simulink model "simulation"  (R2018a)
settings: Solver=VariableStepAuto  StartTime=0.0  StopTime=5  RelTol=1e-3
libraries: simulink x3, vrlib x1
settings Model: Creator=Juan  LastModifiedBy=Juan

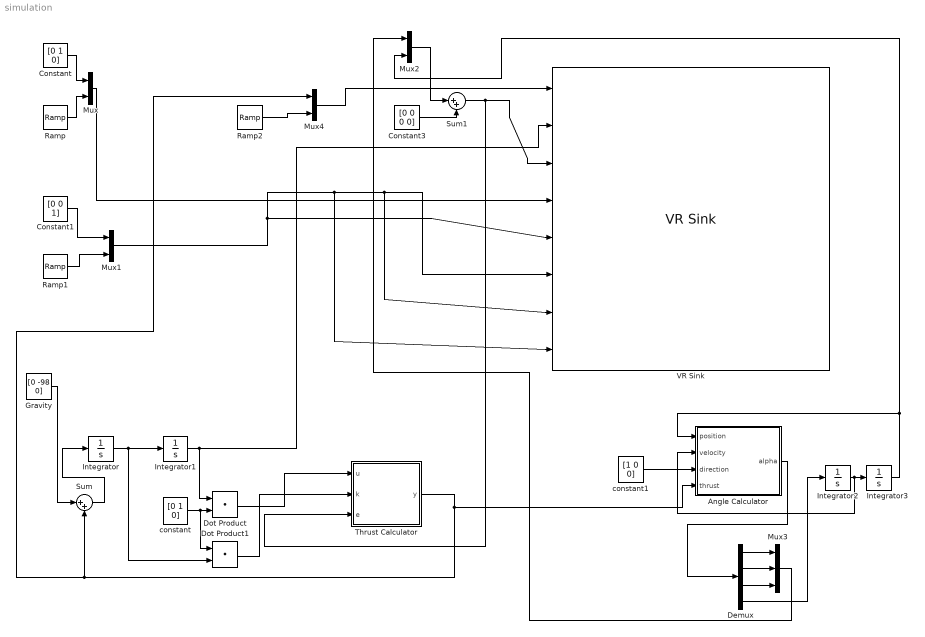
== system simulation ==
  Angle Calculator : MATLAB Function  TreatAsAtomicUnit=on
  Constant : Constant  Value=[0 1 0]  VectorParams1D=off
  Constant1 : Constant  Value=[0 0 1]  VectorParams1D=off
  Constant3 : Constant  Value=[0 0 0 0]  VectorParams1D=off
  Demux : Demux
  Dot Product : DotProduct  InputSameDT=on  OutDataTypeStr=Inherit: Inherit via internal rule
  Dot Product1 : DotProduct  InputSameDT=on  OutDataTypeStr=Inherit: Inherit via internal rule
  Gravity : Constant  Value=[0 -98 0]
  Integrator{,1..3} (4 alike) : Integrator
  Mux{,1..2,4} (4 alike) : Mux  Inputs=2
  Mux3 : Mux  Inputs=3
  Ramp : simulink/Sources/Ramp  slope=10  start=0  InitialOutput=0
  Ramp1 : simulink/Sources/Ramp  slope=25  start=0  InitialOutput=0
  Ramp2 : simulink/Sources/Ramp  slope=-1  start=0  InitialOutput=0
  Sum : Sum  Inputs=|++
  Sum1 : Sum  Inputs=|++
  Thrust Calculator : MATLAB Function  TreatAsAtomicUnit=on
  VR Sink : vrlib/VR Sink  InstantiateOnLoad=on  SampleTime=0.02  ViewEnable=on  RemoteChange=off  RemoteView=off  FieldsWritten=Core.rotation.4.1.1.double#Core.translation.3.1.1.double#quadcopter.rotation.4.1.1.double#motor.rotation.4.1.1.double#propeller_1.rotation.4.1.1.double#propeller_2.rotation.4.1.1.double#propeller_3.rotation.4.1.1.double#propeller_4.rotation.4.1.1.double  WorldFileName=multiView.wrl  AutoView=off  VideoDimensions=[]  AllowVariableSize=off
      settings: SourceProductBaseCode=VR
  constant : Constant  Value=[0 1 0]
  constant1 : Constant  Value=[1 0 0]
  wires:
  Integrator/1 -> Dot Product1/2, Integrator1/1
  Constant/1 -> Mux/1
  Constant1/1 -> Mux1/1
  Ramp1/1 -> Mux1/2
  Sum/1 -> Integrator/1
  Dot Product/1 -> Thrust Calculator/1(u)
  constant/1 -> Dot Product1/1, Dot Product/2
  Dot Product1/1 -> Thrust Calculator/2(k)
  Gravity/1 -> Sum/1
  Thrust Calculator/1(y) -> Mux4/1, Sum/2, Angle Calculator/4(thrust)
  Integrator2/1 -> Angle Calculator/2(velocity), Integrator3/1
  constant1/1 -> Angle Calculator/3(direction)
  Integrator1/1 -> Dot Product/1, VR Sink/2
  Demux/4 -> Integrator2/1
  Demux/1 -> Mux3/1
  Demux/2 -> Mux3/2
  Demux/3 -> Mux3/3
  Mux3/1 -> Mux2/1
  Angle Calculator/1(alpha) -> Demux/1
  Integrator3/1 -> Angle Calculator/1(position), Mux2/2
  Constant3/1 -> Sum1/2
  Mux2/1 -> Sum1/1
  Sum1/1 -> Thrust Calculator/3(e), VR Sink/3
  Mux/1 -> VR Sink/4
  Mux1/1 -> VR Sink/5, VR Sink/6, VR Sink/7, VR Sink/8
  Ramp2/1 -> Mux4/2
  Mux4/1 -> VR Sink/1
  Ramp/1 -> Mux/2

== matlab function simulation/Angle Calculator ==
  data: position input; velocity input; direction input; alpha output; thrust input
function alpha = fcn(position,velocity,direction,thrust)
a=cross(direction,thrust);
b=((dot(a,a)).^0.5)/10;
 if position>=(-pi/8.2)
    b=-b;
 elseif position<=(-pi/8)
    b=b;
 elseif velocity>0
    b=b;
 else
    b=-b;
 end
alpha=[a(1) a(2) abs(a(3)) b];   
end

== matlab function simulation/Thrust Calculator ==
  data: u input; y output; k input; e input
function y = fcn(u,k,e)
    y=[0 120 0];    
    theta=e(4);
    e0=[e(1) e(2) e(3)];
    norm=(dot(e0,e0)).^0.5;
    if norm~=0
    e0=e0./norm;
    end
    y=cos(theta).*y+sin(theta).*cross(e0,y)+(1-cos(theta)).*dot(e0,y).*e0;
end
